simulink model "first_model"  (R2020a)
settings: Solver=FixedStepAuto  StartTime=0.0  StopTime=10.0  RelTol=1e-3
model workspace (MAT data in the model file):
  J = Simulink.Parameter
  J.DataType = 'auto'
  J.Dimensions = [0 0]
undefined symbols (not defined in the file): B, Km, L, R
libraries: simulink x1
settings Model: Creator=utente  LastModifiedBy=utente
settings OptimizationCC: DefaultParameterBehavior=Inlined  UseDivisionForNetSlopeComputation=on  GainParamInheritBuiltInType=on  UseFloatMulNetSlope=on  InlineInvariantSignals=on  EfficientFloat2IntCast=on  LifeSpan=1
settings HardwareCC: ProdBitPerInt=16  ProdBitPerPointer=16  ProdBitPerSizeT=16  ProdBitPerPtrDiffT=16  ProdLargestAtomicFloat=None  ProdWordSize=16  ProdHWDeviceType=Atmel->AVR (8-bit)
settings SFSimCC: MATLABDynamicMemAlloc=off
settings RTWCC: GenerateReport=on  LaunchReport=on
settings CodeAppCC: ForceParamTrailComments=on
settings GRTTargetCC: CombineSignalStateStructs=on  MatFileLogging=off  SupportVariableSizeSignals=on

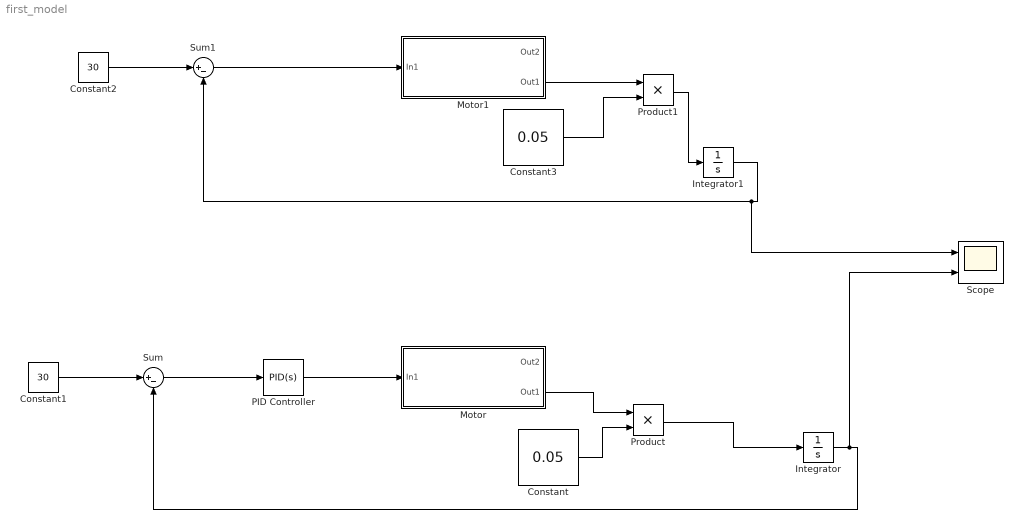
== system first_model ==
  Constant : Constant  Value=0.05  VectorParams1D=off
  Constant1 : Constant  Value=30
  Constant2 : Constant  Value=30
  Constant3 : Constant  Value=0.05  VectorParams1D=off
  Integrator : Integrator
  Integrator1 : Integrator
  Motor : Subsystem
  Motor1 : Subsystem
  PID Controller : simulink/Continuous/PID Controller  Controller=PID  Form=Parallel  TimeDomain=Continuous-time  UseExternalTs=off  SampleTime=-1  IntegratorMethod=Forward Euler  FilterMethod=Forward Euler  ControllerParametersSource=internal  P=900  I=388.285336673823  D=313.362525915555  UseFilter=on  N=12.9901005705061  TunerSelectOption=Transfer Function Based (PID Tuner App)  InitialConditionSource=internal  InitialConditionForIntegrator=0  InitialConditionForFilter=0  DifferentiatorICPrevScaledInput=0  ExternalReset=none  TrackingMode=off  Kt=1  LimitOutput=on  UpperSaturationLimit=1500  LowerSaturationLimit=-inf  LinearizeAsGain=off  AntiWindupMode=clamping  Kb=1  POutMin=[]  POutMax=[]  IOutMin=[]  IOutMax=[]  DOutMin=[]  DOutMax=[]  NOutMin=[]  NOutMax=[]  SumOutMin=[]  SumOutMax=[]  SaturationOutMin=[]  SaturationOutMax=[]  PParamMin=[]  PParamMax=[]  IParamMin=[]  IParamMax=[]  DParamMin=[]  DParamMax=[]  NParamMin=[]  NParamMax=[]  KbParamMin=[]  KbParamMax=[]  KtParamMin=[]  KtParamMax=[]  KbOutMin=[]  KbOutMax=[]  KtOutMin=[]  KtOutMax=[]  IntegratorOutMin=[]  IntegratorOutMax=[]  FilterOutMin=[]  FilterOutMax=[]  SumI1OutMin=[]  SumI1OutMax=[]  SumI2OutMin=[]  SumI2OutMax=[]  SumI3OutMin=[]  SumI3OutMax=[]  SumI4OutMin=[]  SumI4OutMax=[]  SumDOutMin=[]  SumDOutMax=[]  DifferentiatorOutMin=[]  DifferentiatorOutMax=[]  FilterDiffOutCoefMin=[]  FilterDiffOutCoefMax=[]  ReciprocalOutMin=[]  ReciprocalOutMax=[]  SumDenOutMin=[]  SumDenOutMax=[]  SumNumOutMin=[]  SumNumOutMax=[]  DivideOutMin=[]  DivideOutMax=[]  UdiffTsProdOutMin=[]  UdiffTsProdOutMax=[]  NTsProdOutMin=[]  NTsProdOutMax=[]  UintegralTsProdOutMin=[]  UintegralTsProdOutMax=[]  UngainTsProdOutMin=[]  UngainTsProdOutMax=[]  IntegratorContinuousStateAttributes=''  IntegratorStateMustResolveToSignalObject=off  IntegratorRTWStateStorageClass=Auto  FilterContinuousStateAttributes=''  FilterStateMustResolveToSignalObject=off  FilterRTWStateStorageClass=Auto  ParallelPVariant=InternalParameters  IdealPVariant=Disabled  IVariant=InternalParameters  DVariant=InternalParameters  IntegratorVariant=Continuous  SatVariant=Enabled  AWVariant=ContClampingParallel  PCopyVariant=Disabled  TRVariant=Disabled  FdbkBlocksVariant=Forward  IdealPFdbkVariant=Disabled  SatFdbkVariant=Disabled  DerivativeFilterVariant=ContFilter  NVariant=InternalParameters  NCopyVariant=Disabled  FilterICVariant=InternalICsFilter  IntegratorICVariant=InternalICs  ExternalResetVariant=Disabled  TRSumVariant=Passthrough  SumFdbkVariant=Disabled  SumVariant=Sum_PID  TsampFilterVariant=InternalTs  TsampNgainVariant=Passthrough  TsampIntegralVariant=Passthrough
  Product : Product
  Product1 : Product
  Scope : Scope  NumInputPorts=2
  Sum : Sum  Inputs=|+-
  Sum1 : Sum  Inputs=|+-
  wires:
  Motor/2(Out1) -> Product/1
  Constant/1 -> Product/2
  Product/1 -> Integrator/1
  Integrator/1 -> Scope/2, Sum/2
  PID Controller/1 -> Motor/1(In1)
  Sum/1 -> PID Controller/1
  Constant1/1 -> Sum/1
  Constant2/1 -> Sum1/1
  Sum1/1 -> Motor1/1(In1)
  Motor1/2(Out1) -> Product1/1
  Constant3/1 -> Product1/2
  Product1/1 -> Integrator1/1
  Integrator1/1 -> Scope/1, Sum1/2

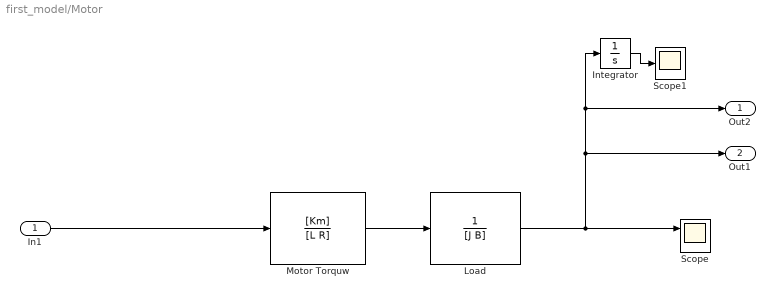
== system first_model/Motor ==
  In1 : Inport
  Integrator : Integrator
  Load : TransferFcn  Denominator=[J B]
  Motor Torquw : TransferFcn  Numerator=[Km]  Denominator=[L R]
  Scope : Scope  NumInputPorts=2
  Scope1 : Scope
  Out2 : Outport
  Out1 : Outport  Port=2
  wires:
  Load/1 -> Scope/1, Out1/1, Out2/1, Integrator/1
  Motor Torquw/1 -> Load/1
  Integrator/1 -> Scope1/1
  In1/1 -> Motor Torquw/1

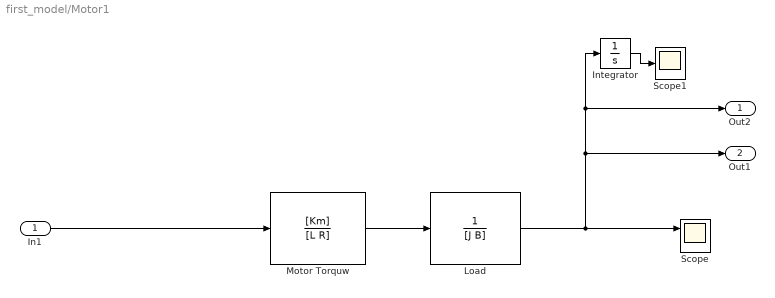
== system first_model/Motor1 ==
  In1 : Inport
  Integrator : Integrator
  Load : TransferFcn  Denominator=[J B]
  Motor Torquw : TransferFcn  Numerator=[Km]  Denominator=[L R]
  Scope : Scope  NumInputPorts=2
  Scope1 : Scope
  Out2 : Outport
  Out1 : Outport  Port=2
  wires:
  Load/1 -> Scope/1, Out1/1, Out2/1, Integrator/1
  Motor Torquw/1 -> Load/1
  Integrator/1 -> Scope1/1
  In1/1 -> Motor Torquw/1
